simulink model "Pacejka1"  (R2020a)
settings: Solver=VariableStepAuto  StartTime=0.0  StopTime=10.0  RelTol=1e-3
undefined symbols (not defined in the file): a0, a1, a10, a11, a12, a13, a2, a3, a4, a5, a6, a7, a8, a9, camber
settings Model: Creator=carmelo  LastModifiedBy=carmelo

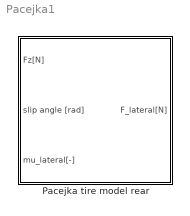
== system Pacejka1 ==
  Pacejka tire model rear : Subsystem

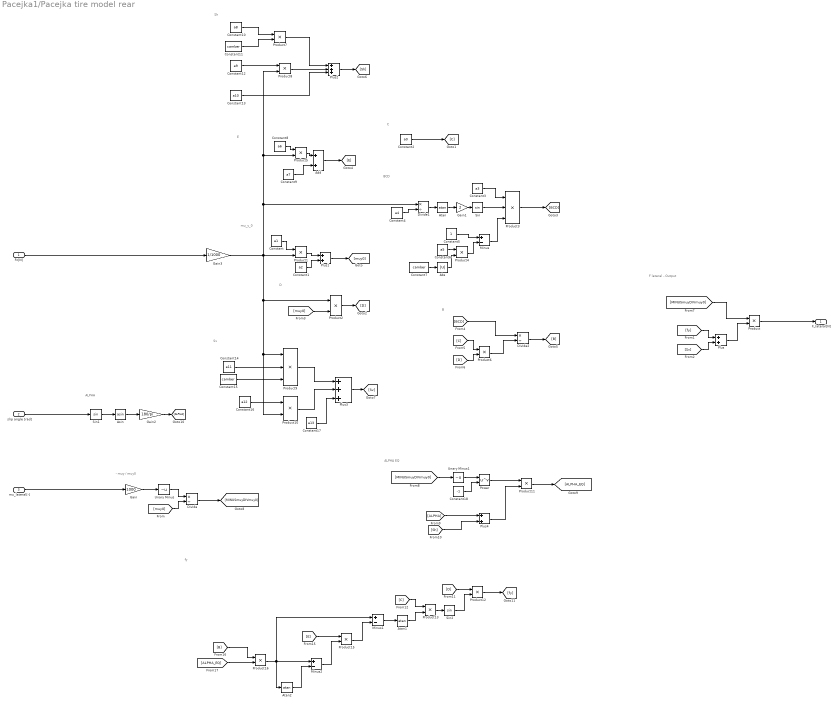
== system Pacejka1/Pacejka tire model rear ==
  note: fy
  note: ALPHA
  note: - muy / muy0
  note: ALPHA EQ
  note: Sv
  note: Sh
  note: B
  note: E
  note: BCD
  note: C
  note: D
  note: mu_y_0
  note: F lateral - Output
  Fz[N] : Inport  Unit=N
  slip angle [rad] : Inport  Port=2  Unit=rad
  mu_lateral[-] : Inport  Port=3
  Abs : Abs
  Add : Sum
  Asin : Trigonometry  Operator=asin
  Atan : Trigonometry  Operator=atan
  Atan1 : Trigonometry  Operator=atan
  Atan2 : Trigonometry  Operator=atan
  Constant : Constant  Value=a1
  Constant1 : Constant  Value=a2
  Constant10 : Constant  Value=a8
  Constant11 : Constant  Value=camber
  Constant12 : Constant  Value=a9
  Constant13 : Constant  Value=a10
  Constant14 : Constant  Value=a11
  Constant15 : Constant  Value=camber
  Constant16 : Constant  Value=a12
  Constant17 : Constant  Value=a13
  Constant18 : Constant  Value=-1
  Constant2 : Constant  Value=a0
  Constant3 : Constant  Value=a3
  Constant4 : Constant  Value=a4
  Constant5 : Constant
  Constant6 : Constant  Value=a5
  Constant7 : Constant  Value=camber
  Constant8 : Constant  Value=a6
  Constant9 : Constant  Value=a7
  Divide : Product  Inputs=*/
  Divide1 : Product  Inputs=*/
  Divide2 : Product  Inputs=*/
  Gain : Gain  Gain=1000
  Gain1 : Gain  Gain=2
  Gain2 : Gain  Gain=180/pi
  Gain3 : Gain  Gain=1/1000
  Minus : Sum  Inputs=+-
  Minus1 : Sum  Inputs=+-
  Minus2 : Sum  Inputs=+-
  Plus : Sum
  Plus1 : Sum
  Plus2 : Sum  Inputs=+++
  Plus3 : Sum  Inputs=+++
  Plus4 : Sum
  Power : Math  Operator=pow  SaturateOnIntegerOverflow=on
  Product{,1..2,4..8,10..13,15..16} (14 alike) : Product
  Product3 : Product  Inputs=3
  Product9 : Product  Inputs=3
  Sin : Trigonometry
  Sin1 : Trigonometry
  Sin2 : Trigonometry
  Unary Minus : UnaryMinus
  Unary Minus1 : UnaryMinus
  F_lateral[N] : Outport  Unit=N
  wires:
  Unary Minus/1 -> Divide/1
  Product7/1 -> Plus2/1
  Sin/1 -> Product3/2
  Constant9/1 -> Add/2
  Asin/1 -> Gain2/1
  Constant8/1 -> Product5/1
  Constant4/1 -> Divide1/2
  Constant10/1 -> Product7/1
  Constant13/1 -> Plus2/3
  Product4/1 -> Minus/2
  [fy] -> Plus/1
  Add/1 -> [E]
  Atan2/1 -> Minus2/2
  Constant3/1 -> Product3/1
  Gain1/1 -> Sin/1
  Sin2/1 -> Product12/2
  Constant15/1 -> Product9/3
  Abs/1 -> Product4/2
  [BCD] -> Divide2/1
  Constant5/1 -> Minus/1
  [D] -> Product12/1
  Product2/1 -> [D]
  Constant6/1 -> Product4/1
  [Sv] -> Plus/2
  Divide1/1 -> Atan/1
  Product8/1 -> Plus2/2
  Fz[N]/1 -> Gain3/1
  Product16/1 -> Minus1/1, Atan2/1, Minus2/1
  Sin1/1 -> Asin/1
  Plus4/1 -> Product11/2
  [C] -> Product6/1
  Product3/1 -> [BCD]
  Product9/1 -> Plus3/1
  Constant17/1 -> Plus3/3
  Product6/1 -> Divide2/2
  Product13/1 -> Sin2/1
  Gain2/1 -> [ALPHA]
  Product12/1 -> [fy]
  Plus2/1 -> [Sh]
  Plus1/1 -> [muy0]
  mu_lateral[-]/1 -> Gain/1
  [ALPHA_EQ] -> Product16/2
  Product10/1 -> Plus3/2
  [MINUSmuyDIVmuy0] -> Product/1
  [muy0] -> Product2/2
  [ALPHA] -> Plus4/1
  [D] -> Product6/2
  Constant/1 -> Product1/1
  Gain3/1 -> Divide1/1, Product5/2, Product8/2, Product1/2, Product2/1, Product9/1, Product10/2
  Unary Minus1/1 -> Power/1
  Constant18/1 -> Power/2
  Product5/1 -> Add/1
  Minus1/1 -> Atan1/1
  [E] -> Product15/1
  [Sh] -> Plus4/2
  Plus/1 -> Product/2
  Constant11/1 -> Product7/2
  Plus3/1 -> [Sv]
  Product/1 -> F_lateral[N]/1
  Constant1/1 -> Plus1/2
  Power/1 -> Product11/1
  Atan1/1 -> Product13/2
  [muy0] -> Divide/2
  Product15/1 -> Minus1/2
  Constant14/1 -> Product9/2
  Constant2/1 -> [C]
  Divide/1 -> [MINUSmuyDIVmuy0]
  Gain/1 -> Unary Minus/1
  Product11/1 -> [ALPHA_EQ]
  Constant16/1 -> Product10/1
  Atan/1 -> Gain1/1
  Constant7/1 -> Abs/1
  [MINUSmuyDIVmuy0] -> Unary Minus1/1
  Constant12/1 -> Product8/1
  [C] -> Product13/1
  Minus2/1 -> Product15/2
  slip angle [rad]/1 -> Sin1/1
  Divide2/1 -> [B]
  Product1/1 -> Plus1/1
  Minus/1 -> Product3/3
  [B] -> Product16/1
